simulink model "param_tuning"  (R2022a)
settings: Solver=VariableStepAuto  StartTime=0.0  StopTime=10  RelTol=1e-3
model workspace (MAT data in the model file):
  K = Simulink.Parameter
  K.Value = [0.012 0.29]
  K.DataType = 'auto'
  K.Complexity = 'real'
  K.Dimensions = [1 2]
  Kt = Simulink.Parameter
  Kt.Value = 15.7
  Kt.DataType = 'double'
  Kt.Complexity = 'real'
  Kt.Dimensions = [1 1]
libraries: slpidlib x1
settings Model: Creator=fkfk21  LastModifiedBy=fkfk21

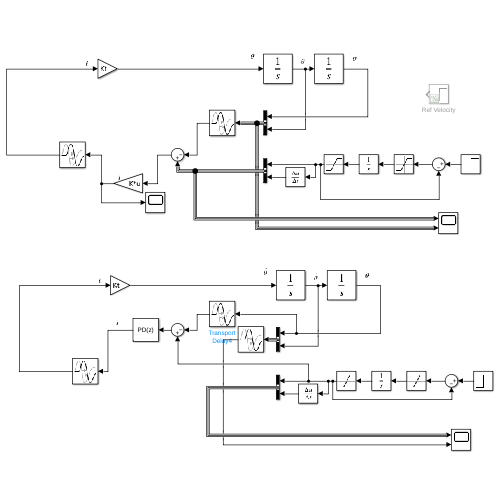
[thumbnail: Simulink's stored preview of the top-level diagram]
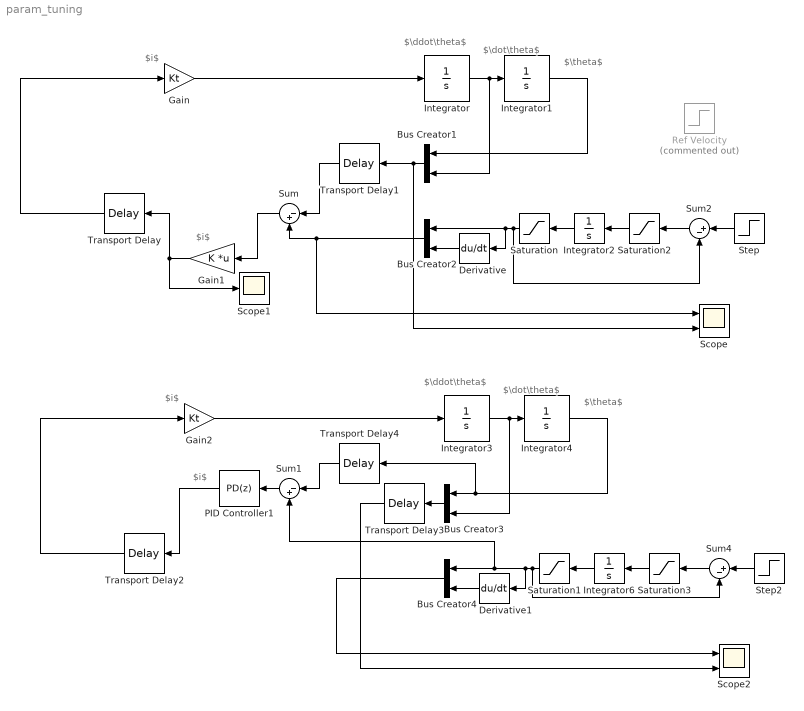
== system param_tuning ==
  note: $i$
  note: $\ddot\theta$
  note: $\dot\theta$
  note: $\theta$
  note: $i$
  note: $\theta$
  note: $\ddot\theta$
  note: $i$
  note: $\dot\theta$
  note: $i$
  Bus Creator{1..4} (4 alike) : BusCreator  Inputs=2
  Derivative : Derivative
  Derivative1 : Derivative
  Gain : Gain  Gain=Kt
  Gain1 : Gain  Gain=K  Multiplication=Matrix(K*u)
  Gain2 : Gain  Gain=Kt
  Integrator{,1..4,6} (6 alike) : Integrator
  PID Controller1 : slpidlib/PID Controller  Controller=PD  Form=Parallel  TimeDomain=Discrete-time  UseExternalTs=off  SampleTime=-1  IntegratorMethod=Forward Euler  FilterMethod=Forward Euler  ControllerParametersSource=internal  P=0.0114421381424435  I=1  UseKiTs=off  D=0.288428415523775  N=83.8208892290339  UseFilter=on  TunerSelectOption=Transfer Function Based (PID Tuner App)  InitialConditionSource=internal  InitialConditionForIntegrator=0  InitialConditionForFilter=0  DifferentiatorICPrevScaledInput=0  ExternalReset=none  TrackingMode=off  Kt=1  LimitOutput=off  SatLimitsSource=internal  UpperSaturationLimit=inf  LowerSaturationLimit=-inf  LinearizeAsGain=on  AntiWindupMode=none  Kb=1  POutMin=[]  POutMax=[]  IOutMin=[]  IOutMax=[]  DOutMin=[]  DOutMax=[]  NOutMin=[]  NOutMax=[]  SumOutMin=[]  SumOutMax=[]  SaturationOutMin=[]  SaturationOutMax=[]  PParamMin=[]  PParamMax=[]  IParamMin=[]  IParamMax=[]  DParamMin=[]  DParamMax=[]  NParamMin=[]  NParamMax=[]  KbParamMin=[]  KbParamMax=[]  KtParamMin=[]  KtParamMax=[]  KbOutMin=[]  KbOutMax=[]  KtOutMin=[]  KtOutMax=[]  IntegratorOutMin=[]  IntegratorOutMax=[]  FilterOutMin=[]  FilterOutMax=[]  SumI1OutMin=[]  SumI1OutMax=[]  SumI2OutMin=[]  SumI2OutMax=[]  SumI3OutMin=[]  SumI3OutMax=[]  SumI4OutMin=[]  SumI4OutMax=[]  SumDOutMin=[]  SumDOutMax=[]  DifferentiatorOutMin=[]  DifferentiatorOutMax=[]  FilterDiffOutCoefMin=[]  FilterDiffOutCoefMax=[]  ReciprocalOutMin=[]  ReciprocalOutMax=[]  SumDenOutMin=[]  SumDenOutMax=[]  SumNumOutMin=[]  SumNumOutMax=[]  DivideOutMin=[]  DivideOutMax=[]  UdiffTsProdOutMin=[]  UdiffTsProdOutMax=[]  NTsProdOutMin=[]  NTsProdOutMax=[]  UintegralTsProdOutMin=[]  UintegralTsProdOutMax=[]  UngainTsProdOutMin=[]  UngainTsProdOutMax=[]  IntegratorContinuousStateAttributes=''  IntegratorStateMustResolveToSignalObject=off  IntegratorRTWStateStorageClass=Auto  FilterContinuousStateAttributes=''  FilterStateMustResolveToSignalObject=off  FilterRTWStateStorageClass=Auto  ParallelPVariant=InternalParameters  IdealPVariant=Disabled  IVariant=Disabled  DVariant=InternalParameters  IntegratorVariant=Disabled  SatVariant=Disabled  AWVariant=Disabled  PCopyVariant=Disabled  TRVariant=Disabled  FdbkBlocksVariant=Forward  IdealPFdbkVariant=Disabled  SatFdbkVariant=Disabled  DerivativeFilterVariant=ForwardEulerFilter  NVariant=InternalParameters  NCopyVariant=Disabled  FilterICVariant=InternalICsFilter  IntegratorICVariant=Disabled  ExternalResetVariant=Disabled  TRSumVariant=Passthrough  SumFdbkVariant=Disabled  SumVariant=Sum_PD  TsampFilterVariant=InternalTs  TsampNgainVariant=Passthrough  TsampIntegralVariant=Disabled_SignalSpec  ExternalSaturationOutDataTypeStr=Inherit: Same as second input  aMode=0
  Ref Velocity : Step  Commented=on  Time=0  After=1.5  SampleTime=0.02
  Saturation : Saturate  UpperLimit=5
  Saturation1 : Saturate  UpperLimit=5
  Saturation2 : Saturate  UpperLimit=3  LowerLimit=-3
  Saturation3 : Saturate  UpperLimit=3  LowerLimit=-3
  Scope : Scope  NumInputPorts=2
  Scope1 : Scope
  Scope2 : Scope  NumInputPorts=2
  Step : Step  Time=0  After=5  SampleTime=0.02
  Step2 : Step  Time=0  After=5  SampleTime=0.02
  Sum : Sum  Inputs=|-+
  Sum1 : Sum  Inputs=|-+
  Sum2 : Sum  Inputs=|+-
  Sum4 : Sum  Inputs=|+-
  Transport Delay : TransportDelay  DelayTime=0.005
  Transport Delay1 : TransportDelay  DelayTime=0.06
  Transport Delay2 : TransportDelay  DelayTime=0.005
  Transport Delay3 : TransportDelay  DelayTime=0.04
  Transport Delay4 : TransportDelay  DelayTime=0.06
  wires:
  Gain/1 -> Integrator/1
  Integrator/1 -> Bus Creator1/2, Integrator1/1
  Integrator1/1 -> Bus Creator1/1
  Bus Creator1/1 -> Transport Delay1/1, Scope/2
  Transport Delay/1 -> Gain/1
  Integrator2/1 -> Saturation/1
  Saturation/1 -> Sum2/2, Derivative/1, Bus Creator2/1
  Derivative/1 -> Bus Creator2/2
  Sum/1 -> Gain1/1
  Bus Creator2/1 -> Scope/1, Sum/2
  Gain1/1 -> Transport Delay/1, Scope1/1
  Transport Delay1/1 -> Sum/1
  Derivative1/1 -> Bus Creator4/2
  Bus Creator4/1 -> Scope2/1
  Bus Creator3/1 -> Transport Delay3/1
  Integrator4/1 -> Transport Delay4/1, Bus Creator3/1
  Transport Delay2/1 -> Gain2/1
  Gain2/1 -> Integrator3/1
  Integrator3/1 -> Bus Creator3/2, Integrator4/1
  Sum1/1 -> PID Controller1/1
  Transport Delay3/1 -> Scope2/2
  Transport Delay4/1 -> Sum1/1
  PID Controller1/1 -> Transport Delay2/1
  Step/1 -> Sum2/1
  Sum2/1 -> Saturation2/1
  Saturation1/1 -> Sum4/2, Sum1/2, Bus Creator4/1, Derivative1/1
  Saturation2/1 -> Integrator2/1
  Saturation3/1 -> Integrator6/1
  Sum4/1 -> Saturation3/1
  Step2/1 -> Sum4/1
  Integrator6/1 -> Saturation1/1
